simulink model "NolinearObserver"  (R2023b)
settings: Solver=FixedStepDiscrete  StartTime=0.0  StopTime=10  FixedStep=Ts  RelTol=1e-3
values from neighbouring files (symbols this model uses):
  current_bandwidth = 2216.0    [NolinearObserver.sldd]
  flux = 0.0065    [NolinearObserver.sldd]
  Gama = 100000.0    [NolinearObserver.sldd]
  Idq_limit = 10.0    [NolinearObserver.sldd]
  IF_Initial = 30.0    [NolinearObserver.sldd]
  PLL_KI = 20000.0    [NolinearObserver.sldd]
  PLL_KP = 500.0    [NolinearObserver.sldd]
  PMSM_Ls = 8.5E-5    [NolinearObserver.sldd]
  PMSM_Pn = 5.0    [NolinearObserver.sldd]
  PMSM_Rs = 0.03    [NolinearObserver.sldd]
  SPEED_KI = 0.03    [NolinearObserver.sldd]
  SPEED_KP = 0.004    [NolinearObserver.sldd]
  Ts = 0.0001    [NolinearObserver.sldd]
undefined symbols (not defined in the file or in its folder): DiscIntNeverNeededParam
libraries: slpidlib x4, mcbplantlib x1, autolibpmsmexterior x1
settings Model: DataDictionary=NolinearObserver.sldd  NumberOfSteps=50  SnapshotBufferSize=1000  Creator=33595  LastModifiedBy=SkyLin
settings OptimizationCC: DefaultParameterBehavior=Inlined  UseDivisionForNetSlopeComputation=on  GainParamInheritBuiltInType=on  UseFloatMulNetSlope=on  InlineInvariantSignals=on  PassReuseOutputArgsAs=Individual arguments  ZeroExternalMemoryAtStartup=off  ZeroInternalMemoryAtStartup=off  NoFixptDivByZeroProtection=on  EfficientFloat2IntCast=on  LifeSpan=1  OptimizeBlockOrder=speed  DifferentSizesBufferReuse=on  EfficientTunableParamExpr=on
settings DebuggingCC: ParameterOverflowMsg=none  ParameterUnderflowMsg=error  ParameterPrecisionLossMsg=none  ParameterTunabilityLossMsg=error  UnconnectedInputMsg=warning  UnconnectedOutputMsg=warning  UnconnectedLineMsg=warning
settings HardwareCC: ProdBitPerPointer=32  ProdBitPerSizeT=32  ProdBitPerPtrDiffT=32  ProdLargestAtomicInteger=Long  ProdLargestAtomicFloat=Double  ProdWordSize=32  ProdLongLongMode=on  ProdHWDeviceType=ARM Compatible->ARM Cortex-M
settings ModelReferenceCC: EnableRefExpFcnMdlSchedulingChecks=on
settings SFSimCC: MATLABDynamicMemAlloc=off
settings RTWCC: Description=Embedded Coder  SystemTargetFile=ert.tlc  GenCodeOnly=on  TemplateMakefile=ert_default_tmf  RTWUseSimCustomCode=on  DLArmComputeVersion=19.05
settings CodeAppCC: ForceParamTrailComments=on  IgnoreCustomStorageClasses=off  OperatorAnnotations=on  SimulinkDataObjDesc=on  SFDataObjDesc=on  CustomSymbolStrGlobalVar=rt$N$M  CustomSymbolStrType=$N$M  CustomSymbolStrFcn=$N$M$F  CustomSymbolStrMacro=$N$M  InsertBlockDesc=on
settings ERTTargetCC: TargetLangStandard=C99 (ISO)  CodeReplacementLibrary=ARM Cortex-M  GenerateSampleERTMain=on  IncludeMdlTerminateFcn=off  CombineSignalStateStructs=on  SupportComplex=off  SupportNonInlinedSFcns=on  InlinedParameterPlacement=NonHierarchical  ERTCustomFileTemplate=example_file_process.tlc  ERTFilePackagingFormat=CompactWithDataFile  IndentSize=4

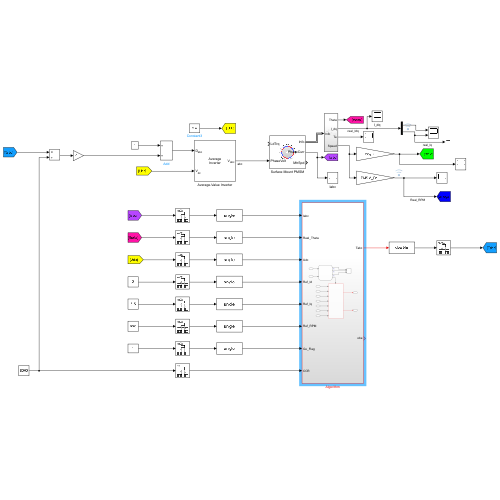
[thumbnail: Simulink's stored preview of the top-level diagram]
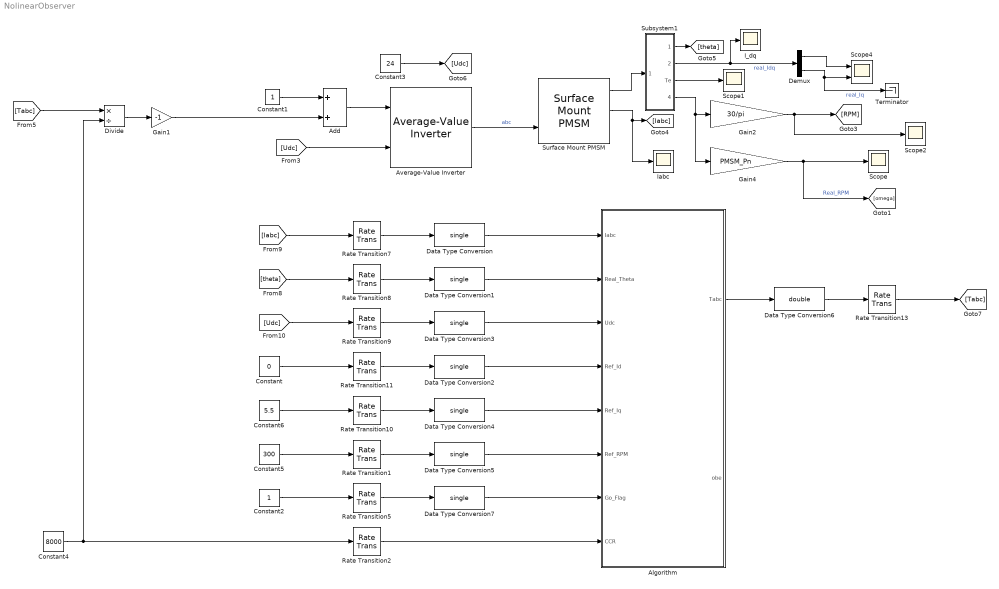
== system NolinearObserver ==
  Add : Sum
  Algorithm : Subsystem
  Average-Value Inverter : mcbplantlib/Average-Value Inverter
  Constant : Constant  Value=0  OutDataTypeStr=single  SampleTime=Ts
  Constant1 : Constant  SampleTime=Ts
  Constant2 : Constant  SampleTime=-1
  Constant3 : Constant  Value=24  SampleTime=Ts
  Constant4 : Constant  Value=8000
  Constant5 : Constant  Value=300
  Constant6 : Constant  Value=5.5
  Data Type Conversion{,1..5,7} (7 alike) : DataTypeConversion  OutDataTypeStr=single  SaturateOnIntegerOverflow=off  RndMeth=Floor
  Data Type Conversion6 : DataTypeConversion  OutDataTypeStr=double  SaturateOnIntegerOverflow=off  RndMeth=Floor
  Demux : Demux  Outputs=2
  Divide : Product  Inputs=*/
  Gain1 : Gain  Gain=-1
  Gain2 : Gain  Gain=30/pi
  Gain4 : Gain  Gain=PMSM_Pn
  I_dq : Scope
  Iabc : Scope
  Rate Transition{1..2,5,8..11,13} (8 alike) : RateTransition  OutPortSampleTime=Ts
  Rate Transition7 : RateTransition
  Scope : Scope
  Scope1 : Scope
  Scope2 : Scope
  Scope4 : Scope  NumInputPorts=2
  Subsystem1 : Subsystem
  Surface Mount PMSM : autolibpmsmexterior/Surface Mount PMSM  port_config=Torque  sim_type=Discrete  Ts=Ts  P=PMSM_Pn  Rs=PMSM_Rs  Ldq_=PMSM_Ls  KConstText=Permanent flux linkage constant (lambda_pm):  lambda_pm=PMSM_flux  Ke=159.9771  Kt=1.323  mechanical=[0.0027, 0.0065, 0]  idq0=[0 0]  theta_init=1  omega_init=0  KConst=PMSM_flux  lambda_pm_calc=PMSM_flux  RefBlkName='autolibpmsmexterior/Surface Mount PMSM'  aMode=5  Ldq="[0.0017      0.0017]"
  Terminator : Terminator
  wires:
  Constant3/1 -> [Udc]
  Subsystem1/1(Theta) -> [theta]
  Subsystem1/2(I_dq) -> Demux/1, I_dq/1  "real_Idq"
  Subsystem1/3(Te) -> Scope1/1
  Subsystem1/4(Speed) -> Gain4/1, Gain2/1
  Average-Value Inverter/1 -> Surface Mount PMSM/2  "abc"
  Surface Mount PMSM/1 -> Subsystem1/1(Info)
  Surface Mount PMSM/2 -> Iabc/1, [Iabc]
  [Udc] -> Average-Value Inverter/2
  Gain2/1 -> Scope2/1, [RPM]
  Gain4/1 -> [omega], Scope/1  "Real_RPM"
  Demux/2 -> Scope4/2, Terminator/1  "real_Iq"
  Data Type Conversion2/1 -> Algorithm/4(Ref_Id)
  [Udc] -> Rate Transition9/1
  Rate Transition13/1 -> [Tabc]
  [Iabc] -> Rate Transition7/1
  Rate Transition10/1 -> Data Type Conversion4/1
  Algorithm/1(Tabc) -> Data Type Conversion6/1
  Data Type Conversion1/1 -> Algorithm/2(Real_Theta)
  Data Type Conversion/1 -> Algorithm/1(Iabc)
  Rate Transition11/1 -> Data Type Conversion2/1
  [theta] -> Rate Transition8/1
  Rate Transition7/1 -> Data Type Conversion/1
  Data Type Conversion6/1 -> Rate Transition13/1
  Rate Transition8/1 -> Data Type Conversion1/1
  Constant/1 -> Rate Transition11/1
  Data Type Conversion4/1 -> Algorithm/5(Ref_Iq)
  Rate Transition9/1 -> Data Type Conversion3/1
  Data Type Conversion3/1 -> Algorithm/3(Udc)
  Add/1 -> Average-Value Inverter/1
  Constant1/1 -> Add/1
  Demux/1 -> Scope4/1
  Rate Transition1/1 -> Data Type Conversion5/1
  Data Type Conversion5/1 -> Algorithm/6(Ref_RPM)
  Constant2/1 -> Rate Transition5/1
  Rate Transition5/1 -> Data Type Conversion7/1
  Data Type Conversion7/1 -> Algorithm/7(Go_Flag)
  Constant6/1 -> Rate Transition10/1
  Constant5/1 -> Rate Transition1/1
  Constant4/1 -> Divide/2, Rate Transition2/1
  Divide/1 -> Gain1/1
  [Tabc] -> Divide/1
  Gain1/1 -> Add/2
  Rate Transition2/1 -> Algorithm/8(CCR)

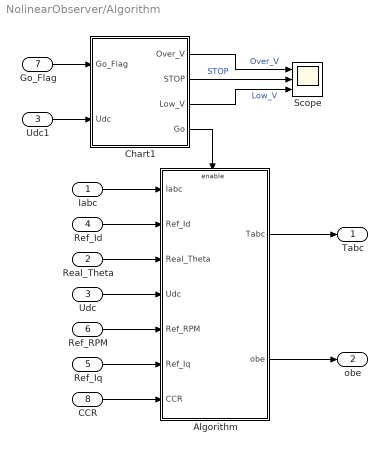
== system NolinearObserver/Algorithm ==
  Iabc : Inport  OutDataTypeStr=single
  Real_Theta : Inport  Port=2  OutDataTypeStr=single
  Udc : Inport  Port=3  OutDataTypeStr=single
  Ref_Id : Inport  Port=4  OutDataTypeStr=single
  Ref_Iq : Inport  Port=5  OutDataTypeStr=single
  Ref_RPM : Inport  Port=6
  Go_Flag : Inport  Port=7
  CCR : Inport  Port=8
  Algorithm : Subsystem
  Chart1 : Stateflow chart  TreatAsAtomicUnit=on
  Scope : Scope  NumInputPorts=3
  Udc1 : InportShadow  Port=3  OutDataTypeStr=single
  Tabc : Outport  OutDataTypeStr=single
  obe : Outport  Port=2
  wires:
  Iabc/1 -> Algorithm/1(Iabc)
  Ref_Id/1 -> Algorithm/2(Ref_Id)
  Real_Theta/1 -> Algorithm/3(Real_Theta)
  Udc/1 -> Algorithm/4(Udc)
  Ref_RPM/1 -> Algorithm/5(Ref_RPM)
  Ref_Iq/1 -> Algorithm/6(Ref_Iq)
  Algorithm/1(Tabc) -> Tabc/1
  Chart1/1(Over_V) -> Scope/1  "Over_V"
  Chart1/2(STOP) -> Scope/2  "STOP"
  Chart1/3(Low_V) -> Scope/3  "Low_V"
  Udc1/1 -> Chart1/2(Udc)
  Go_Flag/1 -> Chart1/1(Go_Flag)
  Chart1/4(Go) -> Algorithm/Enable
  Algorithm/2(obe) -> obe/1
  CCR/1 -> Algorithm/7(CCR)

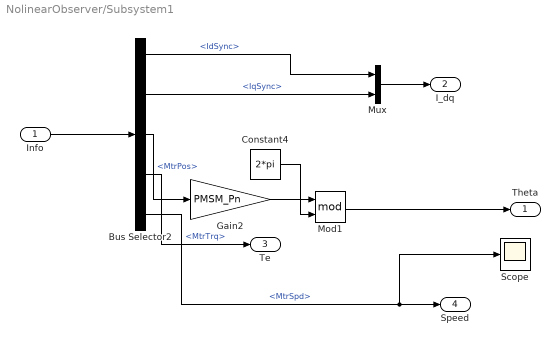
== system NolinearObserver/Subsystem1 ==
  Info : Inport
  Bus Selector2 : BusSelector  OutputSignals=IdSync,IqSync,MtrPos,MtrTrq,MtrSpd
  Constant4 : Constant  Value=2*pi  SampleTime=-1
  Gain2 : Gain  Gain=PMSM_Pn
  Mod1 : Math  Operator=mod
  Mux : Mux  Inputs=2
  Scope : Scope
  Theta : Outport
  I_dq : Outport  Port=2
  Te : Outport  Port=3
  Speed : Outport  Port=4
  wires:
  Bus Selector2/2 -> Mux/2  "<IqSync>"
  Gain2/1 -> Mod1/1
  Mod1/1 -> Theta/1
  Bus Selector2/1 -> Mux/1  "<IdSync>"
  Constant4/1 -> Mod1/2
  Info/1 -> Bus Selector2/1
  Bus Selector2/3 -> Gain2/1  "<MtrPos>"
  Mux/1 -> I_dq/1
  Bus Selector2/4 -> Te/1  "<MtrTrq>"
  Bus Selector2/5 -> Scope/1, Speed/1  "<MtrSpd>"

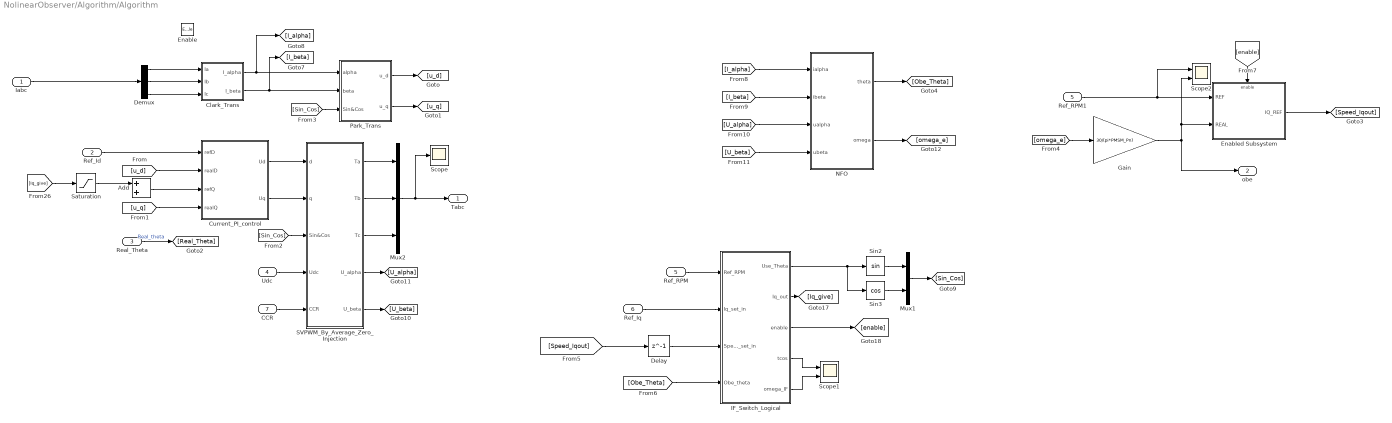
== system NolinearObserver/Algorithm/Algorithm ==
  Iabc : Inport
  Ref_Id : Inport  Port=2
  Real_Theta : Inport  Port=3
  Udc : Inport  Port=4
  Ref_RPM : Inport  Port=5
  Ref_Iq : Inport  Port=6
  CCR : Inport  Port=7
  Enable : EnablePort
  Add : Sum  OutDataTypeStr=single
  Clark_Trans : Subsystem  TreatAsAtomicUnit=on
      settings: RTWFcnNameOpts=Use subsystem name
  Current_PI_control : Subsystem  TreatAsAtomicUnit=on
      settings: RTWFcnNameOpts=Use subsystem name
  Delay : Delay  DelayLength=1
  Demux : Demux  Outputs=3
  Enabled Subsystem : Subsystem  TreatAsAtomicUnit=on
  Gain : Gain  Gain=30/(pi*PMSM_Pn)
  IF_Switch_Logical : Stateflow chart  TreatAsAtomicUnit=on
  Mux1 : Mux  Inputs=2
  Mux2 : Mux  Inputs=3
  NFO : Subsystem
  Park_Trans : Subsystem  TreatAsAtomicUnit=on
      settings: RTWFcnNameOpts=Use subsystem name
  Ref_RPM1 : InportShadow  Port=5
  SVPWM_By_Average_Zero_Injection : Subsystem  TreatAsAtomicUnit=on
  Saturation : Saturate  UpperLimit=Idq_limit  LowerLimit=-Idq_limit  OutDataTypeStr=single
  Scope : Scope
  Scope1 : Scope  NumInputPorts=2
  Scope2 : Scope  NumInputPorts=2
  Sin2 : Trigonometry
  Sin3 : Trigonometry  Operator=cos
  Tabc : Outport
  obe : Outport  Port=2
  wires:
  Sin3/1 -> Mux1/2
  Sin2/1 -> Mux1/1
  Add/1 -> Current_PI_control/3(refQ)
  Iabc/1 -> Demux/1
  [Sin_Cos] -> Park_Trans/3(Sin&Cos)
  Clark_Trans/2(I_beta) -> [I_beta], Park_Trans/2(beta)
  Demux/3 -> Clark_Trans/3(Ic)
  Clark_Trans/1(I_alpha) -> [I_alpha], Park_Trans/1(alpha)
  Park_Trans/2(u_q) -> [u_q]
  SVPWM_By_Average_Zero_Injection/2(Tb) -> Mux2/2
  SVPWM_By_Average_Zero_Injection/3(Tc) -> Mux2/3
  SVPWM_By_Average_Zero_Injection/1(Ta) -> Mux2/1
  [u_q] -> Current_PI_control/4(realQ)
  Demux/2 -> Clark_Trans/2(Ib)
  [Sin_Cos] -> SVPWM_By_Average_Zero_Injection/3(Sin&Cos)
  SVPWM_By_Average_Zero_Injection/5(U_beta) -> [U_beta]
  Park_Trans/1(u_d) -> [u_d]
  [u_d] -> Current_PI_control/2(realD)
  Demux/1 -> Clark_Trans/1(Ia)
  [Iq_give] -> Saturation/1
  SVPWM_By_Average_Zero_Injection/4(U_alpha) -> [U_alpha]
  Current_PI_control/1(Ud) -> SVPWM_By_Average_Zero_Injection/1(d)
  Saturation/1 -> Add/1
  Mux2/1 -> Scope/1, Tabc/1
  Current_PI_control/2(Uq) -> SVPWM_By_Average_Zero_Injection/2(q)
  Ref_Id/1 -> Current_PI_control/1(refD)
  Mux1/1 -> [Sin_Cos]
  Real_Theta/1 -> [Real_Theta]  "Real_theta"
  Udc/1 -> SVPWM_By_Average_Zero_Injection/4(Udc)
  Ref_RPM/1 -> IF_Switch_Logical/1(Ref_RPM)
  IF_Switch_Logical/1(Use_Theta) -> Sin3/1, Sin2/1
  Ref_Iq/1 -> IF_Switch_Logical/2(Iq_set_in)
  IF_Switch_Logical/2(Iq_out) -> [Iq_give]
  IF_Switch_Logical/3(enable) -> [enable]
  IF_Switch_Logical/4(tcos) -> Scope1/1
  IF_Switch_Logical/5(omega_IF) -> Scope1/2
  Enabled Subsystem/1(IQ_REF) -> [Speed_Iqout]
  [enable] -> Enabled Subsystem/Enable
  Ref_RPM1/1 -> Scope2/1, Enabled Subsystem/1(REF)
  Gain/1 -> Scope2/2, Enabled Subsystem/2(REAL), obe/1
  CCR/1 -> SVPWM_By_Average_Zero_Injection/5(CCR)
  [I_alpha] -> NFO/1(ialpha)
  [I_beta] -> NFO/2(ibeta)
  [U_alpha] -> NFO/3(ualpha)
  [U_beta] -> NFO/4(ubeta)
  [omega_e] -> Gain/1
  [Obe_Theta] -> IF_Switch_Logical/4(Obe_theta)
  [Speed_Iqout] -> Delay/1
  Delay/1 -> IF_Switch_Logical/3(Speed_set_in)
  NFO/1(theta) -> [Obe_Theta]
  NFO/2(omega) -> [omega_e]

== system NolinearObserver/Algorithm/Chart1/Low_judge ==
  Input : Inport  OutDataTypeStr=single  PortDimensions=1
  f : TriggerPort  TriggerType=function-call  VariantControl=(inherit)
      settings: CopyFcn=Stateflow.SLINSF.SimulinkMan.removeBlockPreDeleteFcn  PreDeleteFcn=Stateflow.SLINSF.SimulinkMan.unsafePredeleteFcn
  Data Type Conversion : DataTypeConversion  OutDataTypeStr=boolean  SaturateOnIntegerOverflow=off  RndMeth=Floor
  Data Type Conversion1 : DataTypeConversion  OutDataTypeStr=single  SaturateOnIntegerOverflow=off  RndMeth=Floor
  NOR : Logic  Operator=NOT  IconShape=distinctive  OutDataTypeStr=boolean
  Relay : Relay  OnSwitchValue=20  OffSwitchValue=18  OutDataTypeStr=single
  Out : Outport  OutDataTypeStr=single
  wires:
  Input/1 -> Relay/1
  Relay/1 -> Data Type Conversion/1
  NOR/1 -> Data Type Conversion1/1
  Data Type Conversion/1 -> NOR/1
  Data Type Conversion1/1 -> Out/1

== system NolinearObserver/Algorithm/Chart1/Over_judge ==
  Input : Inport  OutDataTypeStr=single  PortDimensions=1
  f : TriggerPort  TriggerType=function-call  VariantControl=(inherit)
      settings: CopyFcn=Stateflow.SLINSF.SimulinkMan.removeBlockPreDeleteFcn  PreDeleteFcn=Stateflow.SLINSF.SimulinkMan.unsafePredeleteFcn
  Relay : Relay  OnSwitchValue=28  OffSwitchValue=25  OutDataTypeStr=single
  Out : Outport  OutDataTypeStr=single
  wires:
  Input/1 -> Relay/1
  Relay/1 -> Out/1

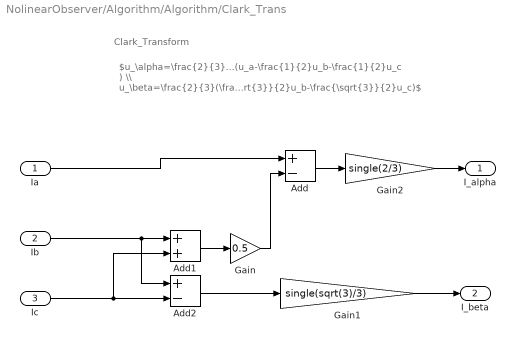
== system NolinearObserver/Algorithm/Algorithm/Clark_Trans ==
  note: $u_\alpha=\frac{2}{3}(u_a-\frac{1}{2}u_b-\frac{1}{2}u_c ) \\ u_\beta=\frac{2}{3}(\frac{\sqrt{3}}{2}u_b-\frac{\sqrt{3}}{2}u_c)$
  note: Clark_Transform
  Ia : Inport  OutDataTypeStr=single
  Ib : Inport  Port=2  OutDataTypeStr=single
  Ic : Inport  Port=3  OutDataTypeStr=single
  Add : Sum  Inputs=+-  OutDataTypeStr=single
  Add1 : Sum  OutDataTypeStr=single
  Add2 : Sum  Inputs=+-  OutDataTypeStr=single
  Gain : Gain  Gain=0.5  OutDataTypeStr=single
  Gain1 : Gain  Gain=single(sqrt(3)/3)  OutDataTypeStr=single
  Gain2 : Gain  Gain=single(2/3)  OutDataTypeStr=single
  I_alpha : Outport  OutDataTypeStr=single
  I_beta : Outport  Port=2
  wires:
  Ia/1 -> Add/1
  Gain/1 -> Add/2
  Ib/1 -> Add1/1, Add2/1
  Ic/1 -> Add1/2, Add2/2
  Add2/1 -> Gain1/1
  Add1/1 -> Gain/1
  Add/1 -> Gain2/1
  Gain2/1 -> I_alpha/1
  Gain1/1 -> I_beta/1

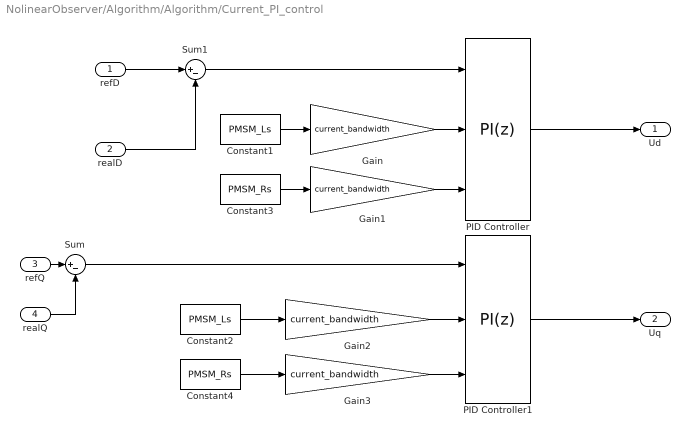
== system NolinearObserver/Algorithm/Algorithm/Current_PI_control ==
  refD : Inport  OutDataTypeStr=single
  realD : Inport  Port=2  OutDataTypeStr=single
  refQ : Inport  Port=3  OutDataTypeStr=single
  realQ : Inport  Port=4  OutDataTypeStr=single
  Constant1 : Constant  Value=PMSM_Ls  OutDataTypeStr=single  SampleTime=Ts
  Constant2 : Constant  Value=PMSM_Ls  OutDataTypeStr=single  SampleTime=Ts
  Constant3 : Constant  Value=PMSM_Rs  OutDataTypeStr=single  SampleTime=Ts
  Constant4 : Constant  Value=PMSM_Rs  OutDataTypeStr=single  SampleTime=Ts
  Gain{,1..3} (4 alike) : Gain  Gain=current_bandwidth  OutDataTypeStr=single
  PID Controller : slpidlib/PID Controller  Controller=PI  Form=Parallel  TimeDomain=Discrete-time  UseExternalTs=off  SampleTime=Ts  IntegratorMethod=Forward Euler  FilterMethod=Forward Euler  ControllerParametersSource=external  P=1  I=1  UseKiTs=off  D=0  N=100  UseFilter=on  TunerSelectOption=Transfer Function Based (PID Tuner App)  ZeroCross=off  InitialConditionSource=internal  InitialConditionForIntegrator=0  InitialConditionForFilter=0  DifferentiatorICPrevScaledInput=0  ExternalReset=none  TrackingMode=off  Kt=1  LimitOutput=on  SatLimitsSource=internal  UpperSaturationLimit=Idq_limit  LowerSaturationLimit=-Idq_limit  LinearizeAsGain=off  AntiWindupMode=none  Kb=1  LimitIntegrator=off  UpperIntegratorSaturationLimit=inf  LowerIntegratorSaturationLimit=-inf  POutMin=[]  POutMax=[]  IOutMin=[]  IOutMax=[]  DOutMin=[]  DOutMax=[]  NOutMin=[]  NOutMax=[]  SumOutMin=[]  SumOutMax=[]  SaturationOutMin=[]  SaturationOutMax=[]  PParamMin=[]  PParamMax=[]  IParamMin=[]  IParamMax=[]  DParamMin=[]  DParamMax=[]  NParamMin=[]  NParamMax=[]  KbParamMin=[]  KbParamMax=[]  KtParamMin=[]  KtParamMax=[]  KbOutMin=[]  KbOutMax=[]  KtOutMin=[]  KtOutMax=[]  IntegratorOutMin=[]  IntegratorOutMax=[]  FilterOutMin=[]  FilterOutMax=[]  SumI1OutMin=[]  SumI1OutMax=[]  SumI2OutMin=[]  SumI2OutMax=[]  SumI3OutMin=[]  SumI3OutMax=[]  SumI4OutMin=[]  SumI4OutMax=[]  SumDOutMin=[]  SumDOutMax=[]  DifferentiatorOutMin=[]  DifferentiatorOutMax=[]  FilterDiffOutCoefMin=[]  FilterDiffOutCoefMax=[]  ReciprocalOutMin=[]  ReciprocalOutMax=[]  SumDenOutMin=[]  SumDenOutMax=[]  SumNumOutMin=[]  SumNumOutMax=[]  DivideOutMin=[]  DivideOutMax=[]  UdiffTsProdOutMin=[]  UdiffTsProdOutMax=[]  NTsProdOutMin=[]  NTsProdOutMax=[]  UintegralTsProdOutMin=[]  UintegralTsProdOutMax=[]  UngainTsProdOutMin=[]  UngainTsProdOutMax=[]  ClampingZeroOutDataTypeStr=Inherit: Inherit via back propagation  ClampingZeroOutMin=[]  ClampingZeroOutMax=[]  FilterDenConstantOutDataTypeStr=Inherit: Inherit via back propagation  FilterDenConstantOutMin=[]  FilterDenConstantOutMax=[]  PCopyOutDataTypeStr=Inherit: Inherit via back propagation  PCopyOutMin=[]  PCopyOutMax=[]  NCopyOutDataTypeStr=Inherit: Inherit via back propagation  NCopyOutMin=[]  NCopyOutMax=[]  IntegratorContinuousStateAttributes=''  IntegratorStateMustResolveToSignalObject=off  IntegratorRTWStateStorageClass=Auto  FilterContinuousStateAttributes=''  FilterStateMustResolveToSignalObject=off  FilterRTWStateStorageClass=Auto  ParallelPVariant=ExternalParameters  IdealPVariant=Disabled  IVariant=ExternalParameters  DVariant=Disabled  IntegratorVariant=Discrete  SatVariant=Enabled  AWVariant=Passthrough  PCopyVariant=Disabled  TRVariant=Disabled  FdbkBlocksVariant=Forward  IdealPFdbkVariant=Disabled  SatFdbkVariant=Disabled  DerivativeFilterVariant=Disabled  NVariant=Disabled  NCopyVariant=Disabled_SignalSpec  FilterICVariant=Disabled  IntegratorICVariant=InternalICs  ExternalResetVariant=Disabled  TRSumVariant=Passthrough  SumFdbkVariant=Disabled  SumVariant=Sum_PI  TsampFilterVariant=InternalTs  TsampNgainVariant=Passthrough  TsampIntegralVariant=Disabled_SignalSpec  ExternalSaturationOutDataTypeStr=Inherit: Same as second input
  PID Controller1 : slpidlib/PID Controller  Controller=PI  Form=Parallel  TimeDomain=Discrete-time  UseExternalTs=off  SampleTime=Ts  IntegratorMethod=Forward Euler  FilterMethod=Forward Euler  ControllerParametersSource=external  P=1  I=1  UseKiTs=off  D=0  N=100  UseFilter=on  TunerSelectOption=Transfer Function Based (PID Tuner App)  ZeroCross=off  InitialConditionSource=internal  InitialConditionForIntegrator=0  InitialConditionForFilter=0  DifferentiatorICPrevScaledInput=0  ExternalReset=none  TrackingMode=off  Kt=1  LimitOutput=on  SatLimitsSource=internal  UpperSaturationLimit=Idq_limit  LowerSaturationLimit=-Idq_limit  LinearizeAsGain=off  AntiWindupMode=none  Kb=1  LimitIntegrator=off  UpperIntegratorSaturationLimit=inf  LowerIntegratorSaturationLimit=-inf  POutMin=[]  POutMax=[]  IOutMin=[]  IOutMax=[]  DOutMin=[]  DOutMax=[]  NOutMin=[]  NOutMax=[]  SumOutMin=[]  SumOutMax=[]  SaturationOutMin=[]  SaturationOutMax=[]  PParamMin=[]  PParamMax=[]  IParamMin=[]  IParamMax=[]  DParamMin=[]  DParamMax=[]  NParamMin=[]  NParamMax=[]  KbParamMin=[]  KbParamMax=[]  KtParamMin=[]  KtParamMax=[]  KbOutMin=[]  KbOutMax=[]  KtOutMin=[]  KtOutMax=[]  IntegratorOutMin=[]  IntegratorOutMax=[]  FilterOutMin=[]  FilterOutMax=[]  SumI1OutMin=[]  SumI1OutMax=[]  SumI2OutMin=[]  SumI2OutMax=[]  SumI3OutMin=[]  SumI3OutMax=[]  SumI4OutMin=[]  SumI4OutMax=[]  SumDOutMin=[]  SumDOutMax=[]  DifferentiatorOutMin=[]  DifferentiatorOutMax=[]  FilterDiffOutCoefMin=[]  FilterDiffOutCoefMax=[]  ReciprocalOutMin=[]  ReciprocalOutMax=[]  SumDenOutMin=[]  SumDenOutMax=[]  SumNumOutMin=[]  SumNumOutMax=[]  DivideOutMin=[]  DivideOutMax=[]  UdiffTsProdOutMin=[]  UdiffTsProdOutMax=[]  NTsProdOutMin=[]  NTsProdOutMax=[]  UintegralTsProdOutMin=[]  UintegralTsProdOutMax=[]  UngainTsProdOutMin=[]  UngainTsProdOutMax=[]  ClampingZeroOutDataTypeStr=Inherit: Inherit via back propagation  ClampingZeroOutMin=[]  ClampingZeroOutMax=[]  FilterDenConstantOutDataTypeStr=Inherit: Inherit via back propagation  FilterDenConstantOutMin=[]  FilterDenConstantOutMax=[]  PCopyOutDataTypeStr=Inherit: Inherit via back propagation  PCopyOutMin=[]  PCopyOutMax=[]  NCopyOutDataTypeStr=Inherit: Inherit via back propagation  NCopyOutMin=[]  NCopyOutMax=[]  IntegratorContinuousStateAttributes=''  IntegratorStateMustResolveToSignalObject=off  IntegratorRTWStateStorageClass=Auto  FilterContinuousStateAttributes=''  FilterStateMustResolveToSignalObject=off  FilterRTWStateStorageClass=Auto  ParallelPVariant=ExternalParameters  IdealPVariant=Disabled  IVariant=ExternalParameters  DVariant=Disabled  IntegratorVariant=Discrete  SatVariant=Enabled  AWVariant=Passthrough  PCopyVariant=Disabled  TRVariant=Disabled  FdbkBlocksVariant=Forward  IdealPFdbkVariant=Disabled  SatFdbkVariant=Disabled  DerivativeFilterVariant=Disabled  NVariant=Disabled  NCopyVariant=Disabled_SignalSpec  FilterICVariant=Disabled  IntegratorICVariant=InternalICs  ExternalResetVariant=Disabled  TRSumVariant=Passthrough  SumFdbkVariant=Disabled  SumVariant=Sum_PI  TsampFilterVariant=InternalTs  TsampNgainVariant=Passthrough  TsampIntegralVariant=Disabled_SignalSpec  ExternalSaturationOutDataTypeStr=Inherit: Same as second input
  Sum : Sum  Inputs=|+-  OutDataTypeStr=single
  Sum1 : Sum  Inputs=|+-  OutDataTypeStr=single
  Ud : Outport  OutDataTypeStr=single
  Uq : Outport  Port=2  OutDataTypeStr=single
  wires:
  realD/1 -> Sum1/2
  realQ/1 -> Sum/2
  PID Controller1/1 -> Uq/1
  PID Controller/1 -> Ud/1
  Sum/1 -> PID Controller1/1
  Sum1/1 -> PID Controller/1
  refD/1 -> Sum1/1
  refQ/1 -> Sum/1
  Constant2/1 -> Gain2/1
  Gain3/1 -> PID Controller1/3
  Gain/1 -> PID Controller/2
  Gain2/1 -> PID Controller1/2
  Constant1/1 -> Gain/1
  Constant4/1 -> Gain3/1
  Gain1/1 -> PID Controller/3
  Constant3/1 -> Gain1/1

== system NolinearObserver/Algorithm/Algorithm/Enabled Subsystem ==
  REF : Inport
  REAL : Inport  Port=2
  Enable : EnablePort
  PID Controller : slpidlib/PID Controller  Controller=PI  Form=Parallel  TimeDomain=Discrete-time  UseExternalTs=off  SampleTime=Ts  IntegratorMethod=Forward Euler  FilterMethod=Forward Euler  ControllerParametersSource=internal  P=SPEED_KP  I=SPEED_KI  UseKiTs=off  D=0  N=100  UseFilter=on  TunerSelectOption=Transfer Function Based (PID Tuner App)  InitialConditionSource=internal  InitialConditionForIntegrator=0  InitialConditionForFilter=0  DifferentiatorICPrevScaledInput=0  ExternalReset=none  TrackingMode=off  Kt=1  LimitOutput=on  SatLimitsSource=internal  UpperSaturationLimit=10  LowerSaturationLimit=-10  LinearizeAsGain=on  AntiWindupMode=none  Kb=1  LimitIntegrator=off  UpperIntegratorSaturationLimit=inf  LowerIntegratorSaturationLimit=-inf  POutMin=[]  POutMax=[]  IOutMin=[]  IOutMax=[]  DOutMin=[]  DOutMax=[]  NOutMin=[]  NOutMax=[]  SumOutMin=[]  SumOutMax=[]  SaturationOutMin=[]  SaturationOutMax=[]  PParamMin=[]  PParamMax=[]  IParamMin=[]  IParamMax=[]  DParamMin=[]  DParamMax=[]  NParamMin=[]  NParamMax=[]  KbParamMin=[]  KbParamMax=[]  KtParamMin=[]  KtParamMax=[]  KbOutMin=[]  KbOutMax=[]  KtOutMin=[]  KtOutMax=[]  IntegratorOutMin=[]  IntegratorOutMax=[]  FilterOutMin=[]  FilterOutMax=[]  SumI1OutMin=[]  SumI1OutMax=[]  SumI2OutMin=[]  SumI2OutMax=[]  SumI3OutMin=[]  SumI3OutMax=[]  SumI4OutMin=[]  SumI4OutMax=[]  SumDOutMin=[]  SumDOutMax=[]  DifferentiatorOutMin=[]  DifferentiatorOutMax=[]  FilterDiffOutCoefMin=[]  FilterDiffOutCoefMax=[]  ReciprocalOutMin=[]  ReciprocalOutMax=[]  SumDenOutMin=[]  SumDenOutMax=[]  SumNumOutMin=[]  SumNumOutMax=[]  DivideOutMin=[]  DivideOutMax=[]  UdiffTsProdOutMin=[]  UdiffTsProdOutMax=[]  NTsProdOutMin=[]  NTsProdOutMax=[]  UintegralTsProdOutMin=[]  UintegralTsProdOutMax=[]  UngainTsProdOutMin=[]  UngainTsProdOutMax=[]  ClampingZeroOutDataTypeStr=Inherit: Inherit via back propagation  ClampingZeroOutMin=[]  ClampingZeroOutMax=[]  FilterDenConstantOutDataTypeStr=Inherit: Inherit via back propagation  FilterDenConstantOutMin=[]  FilterDenConstantOutMax=[]  PCopyOutDataTypeStr=Inherit: Inherit via back propagation  PCopyOutMin=[]  PCopyOutMax=[]  NCopyOutDataTypeStr=Inherit: Inherit via back propagation  NCopyOutMin=[]  NCopyOutMax=[]  IntegratorContinuousStateAttributes=''  IntegratorStateMustResolveToSignalObject=off  IntegratorRTWStateStorageClass=Auto  FilterContinuousStateAttributes=''  FilterStateMustResolveToSignalObject=off  FilterRTWStateStorageClass=Auto  ParallelPVariant=InternalParameters  IdealPVariant=Disabled  IVariant=InternalParameters  DVariant=Disabled  IntegratorVariant=Discrete  SatVariant=Enabled  AWVariant=Passthrough  PCopyVariant=Disabled  TRVariant=Disabled  FdbkBlocksVariant=Forward  IdealPFdbkVariant=Disabled  SatFdbkVariant=Disabled  DerivativeFilterVariant=Disabled  NVariant=Disabled  NCopyVariant=Disabled_SignalSpec  FilterICVariant=Disabled  IntegratorICVariant=InternalICs  ExternalResetVariant=Disabled  TRSumVariant=Passthrough  SumFdbkVariant=Disabled  SumVariant=Sum_PI  TsampFilterVariant=InternalTs  TsampNgainVariant=Passthrough  TsampIntegralVariant=Disabled_SignalSpec  ExternalSaturationOutDataTypeStr=Inherit: Same as second input
  Sum : Sum  Inputs=|+-
  IQ_REF : Outport
  wires:
  REF/1 -> Sum/1
  REAL/1 -> Sum/2
  Sum/1 -> PID Controller/1
  PID Controller/1 -> IQ_REF/1

== system NolinearObserver/Algorithm/Algorithm/IF_Switch_Logical/Forward_theta ==
  direction : Inport  OutDataTypeStr=single  PortDimensions=1
  f : TriggerPort  TriggerType=function-call  VariantControl=(inherit)
      settings: CopyFcn=Stateflow.SLINSF.SimulinkMan.removeBlockPreDeleteFcn  PreDeleteFcn=Stateflow.SLINSF.SimulinkMan.unsafePredeleteFcn
  Constant : Constant  Value=IF_Initial  OutDataTypeStr=single
  Discrete-Time Integrator : DiscreteIntegrator  SampleTime=-1  ICPrevOutput=DiscIntNeverNeededParam  ICPrevScaledInput=DiscIntNeverNeededParam
  Product : Product
  integrator : Subsystem
  IF_theta : Outport  OutDataTypeStr=single
  IF_omega : Outport  Port=2  OutDataTypeStr=single
  wires:
  Constant/1 -> Discrete-Time Integrator/1
  integrator/1(y(k-1)) -> IF_theta/1
  direction/1 -> Product/2
  Discrete-Time Integrator/1 -> Product/1
  Product/1 -> IF_omega/1, integrator/1(x(k))

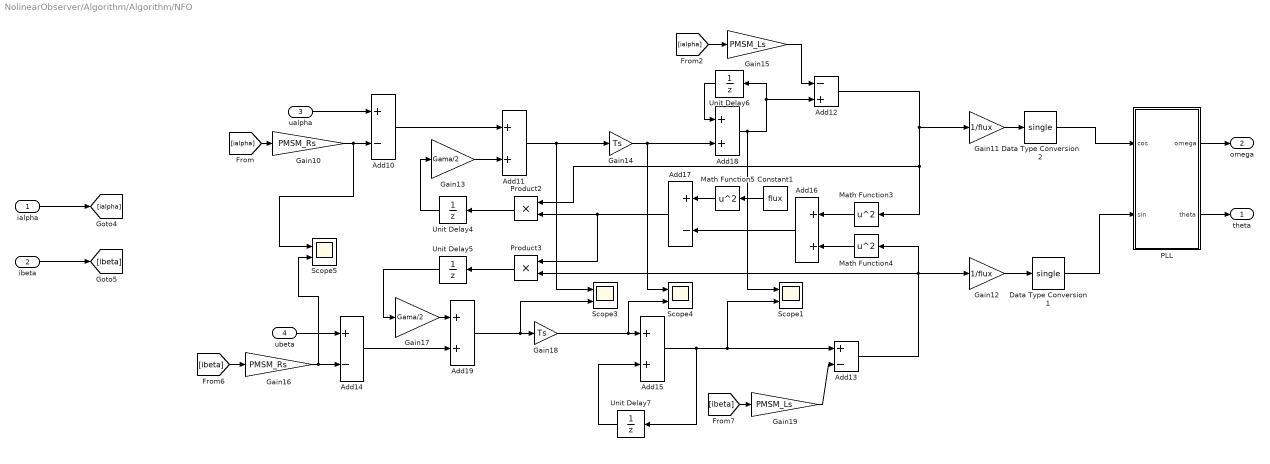
== system NolinearObserver/Algorithm/Algorithm/NFO ==
  ialpha : Inport
  ibeta : Inport  Port=2
  ualpha : Inport  Port=3
  ubeta : Inport  Port=4
  Add{10,13..14,17} (4 alike) : Sum  Inputs=+-
  Add{11,15..16,18..19} (5 alike) : Sum
  Add12 : Sum  Inputs=-+
  Constant1 : Constant  Value=flux
  Data Type Conversion1 : DataTypeConversion  OutDataTypeStr=single  SaturateOnIntegerOverflow=off  RndMeth=Floor
  Data Type Conversion2 : DataTypeConversion  OutDataTypeStr=single  SaturateOnIntegerOverflow=off  RndMeth=Floor
  Gain10 : Gain  Gain=PMSM_Rs
  Gain11 : Gain  Gain=1/flux
  Gain12 : Gain  Gain=1/flux
  Gain13 : Gain  Gain=Gama/2
  Gain14 : Gain  Gain=Ts
  Gain15 : Gain  Gain=PMSM_Ls
  Gain16 : Gain  Gain=PMSM_Rs
  Gain17 : Gain  Gain=Gama/2
  Gain18 : Gain  Gain=Ts
  Gain19 : Gain  Gain=PMSM_Ls
  Math Function3 : Math  Operator=square
  Math Function4 : Math  Operator=square
  Math Function5 : Math  Operator=square
  PLL : Subsystem
  Product2 : Product
  Product3 : Product
  Scope{1,3..5} (4 alike) : Scope  NumInputPorts=2
  Unit Delay{4..7} (4 alike) : UnitDelay  SampleTime=-1  HasFrameUpgradeWarning=on
  theta : Outport  OutDataTypeStr=single
  omega : Outport  Port=2  OutDataTypeStr=single
  wires:
  Gain15/1 -> Add12/1
  Gain17/1 -> Add19/1
  Add17/1 -> Product3/1, Product2/2
  Product3/1 -> Unit Delay5/1
  Add15/1 -> Scope1/2, Add13/1, Unit Delay7/1
  Add19/1 -> Scope3/2, Gain18/1
  [ialpha] -> Gain15/1
  Add13/1 -> Product3/2, Math Function4/1, Gain12/1
  Product2/1 -> Unit Delay4/1
  Gain14/1 -> Scope4/1, Add18/2
  Gain19/1 -> Add13/2
  Add12/1 -> Product2/1, Math Function3/1, Gain11/1
  Unit Delay6/1 -> Add18/1
  ibeta/1 -> [ibeta]
  Gain16/1 -> Scope5/2, Add14/2
  Gain13/1 -> Add11/2
  Add14/1 -> Add19/2
  Unit Delay4/1 -> Gain13/1
  Add10/1 -> Add11/1
  Add16/1 -> Add17/2
  Math Function5/1 -> Add17/1
  [ibeta] -> Gain19/1
  Constant1/1 -> Math Function5/1
  Add18/1 -> Scope1/1, Unit Delay6/1, Add12/2
  Unit Delay7/1 -> Add15/2
  [ibeta] -> Gain16/1
  Math Function4/1 -> Add16/2
  Unit Delay5/1 -> Gain17/1
  Gain18/1 -> Scope4/2, Add15/1
  Add11/1 -> Scope3/1, Gain14/1
  Gain10/1 -> Scope5/1, Add10/2
  Math Function3/1 -> Add16/1
  ialpha/1 -> [ialpha]
  ualpha/1 -> Add10/1
  [ialpha] -> Gain10/1
  ubeta/1 -> Add14/1
  Gain11/1 -> Data Type Conversion2/1
  Gain12/1 -> Data Type Conversion1/1
  Data Type Conversion2/1 -> PLL/1(cos)
  Data Type Conversion1/1 -> PLL/2(sin)
  PLL/1(omega) -> omega/1
  PLL/2(theta) -> theta/1

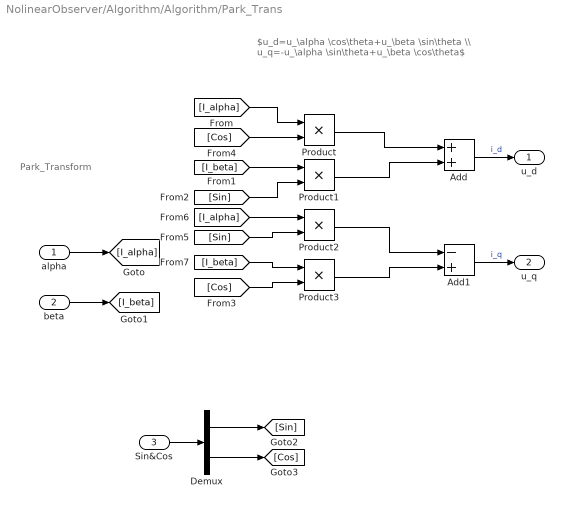
== system NolinearObserver/Algorithm/Algorithm/Park_Trans ==
  note: $u_d=u_\alpha \cos\theta+u_\beta \sin\theta \\ u_q=-u_\alpha \sin\theta+u_\beta \cos\theta$
  note: Park_Transform
  alpha : Inport  OutDataTypeStr=single
  beta : Inport  Port=2  OutDataTypeStr=single
  Sin&Cos : Inport  Port=3  OutDataTypeStr=single
  Add : Sum  OutDataTypeStr=single
  Add1 : Sum  Inputs=-+  OutDataTypeStr=single
  Demux : Demux  Outputs=2
  Product{,1..3} (4 alike) : Product  OutDataTypeStr=single
  u_d : Outport  OutDataTypeStr=single
  u_q : Outport  Port=2  OutDataTypeStr=single
  wires:
  Add1/1 -> u_q/1  "i_q"
  [Cos] -> Product/2
  Product/1 -> Add/1
  Product1/1 -> Add/2
  beta/1 -> [I_beta]
  Add/1 -> u_d/1  "i_d"
  [I_alpha] -> Product/1
  Product3/1 -> Add1/2
  [I_beta] -> Product3/1
  [I_beta] -> Product1/1
  [Sin] -> Product2/2
  Product2/1 -> Add1/1
  [Sin] -> Product1/2
  [I_alpha] -> Product2/1
  alpha/1 -> [I_alpha]
  [Cos] -> Product3/2
  Demux/1 -> [Sin]
  Demux/2 -> [Cos]
  Sin&Cos/1 -> Demux/1

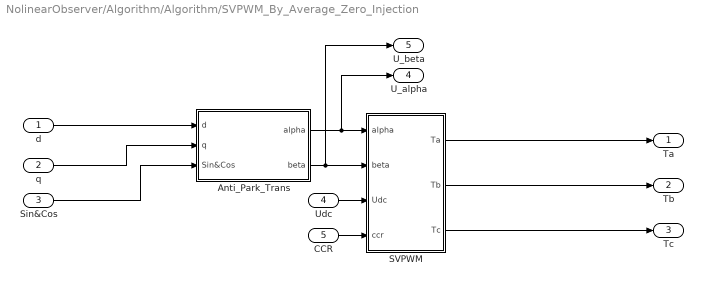
== system NolinearObserver/Algorithm/Algorithm/SVPWM_By_Average_Zero_Injection ==
  d : Inport  OutDataTypeStr=single
  q : Inport  Port=2  OutDataTypeStr=single
  Sin&Cos : Inport  Port=3  OutDataTypeStr=single
  Udc : Inport  Port=4  OutDataTypeStr=single
  CCR : Inport  Port=5
  Anti_Park_Trans : Subsystem
  SVPWM : Subsystem
  Ta : Outport  OutDataTypeStr=single
  Tb : Outport  Port=2  OutDataTypeStr=single
  Tc : Outport  Port=3  OutDataTypeStr=single
  U_alpha : Outport  Port=4  OutDataTypeStr=single
  U_beta : Outport  Port=5  OutDataTypeStr=single
  wires:
  Anti_Park_Trans/1(alpha) -> U_alpha/1, SVPWM/1(alpha)
  q/1 -> Anti_Park_Trans/2(q)
  Anti_Park_Trans/2(beta) -> U_beta/1, SVPWM/2(beta)
  d/1 -> Anti_Park_Trans/1(d)
  Sin&Cos/1 -> Anti_Park_Trans/3(Sin&Cos)
  Udc/1 -> SVPWM/3(Udc)
  SVPWM/1(Ta) -> Ta/1
  SVPWM/2(Tb) -> Tb/1
  SVPWM/3(Tc) -> Tc/1
  CCR/1 -> SVPWM/4(ccr)

== system NolinearObserver/Algorithm/Algorithm/IF_Switch_Logical/Forward_theta/integrator ==
  note: $y(k)=x(k)*T_s+y(k-1)$
  x(k) : Inport  OutDataTypeStr=single
  RangeLimit : Subsystem
  Sum1 : Sum  Inputs=|++  OutDataTypeStr=single
  Ts : Gain  Gain=Ts  OutDataTypeStr=single
  Unit Delay : UnitDelay  SampleTime=-1  HasFrameUpgradeWarning=on
  y(k-1) : Outport  OutDataTypeStr=single
  wires:
  x(k)/1 -> Ts/1
  Ts/1 -> Sum1/1
  Sum1/1 -> RangeLimit/1(In)  "y(k)"
  Unit Delay/1 -> y(k-1)/1, Sum1/2
  RangeLimit/1(Theta) -> Unit Delay/1

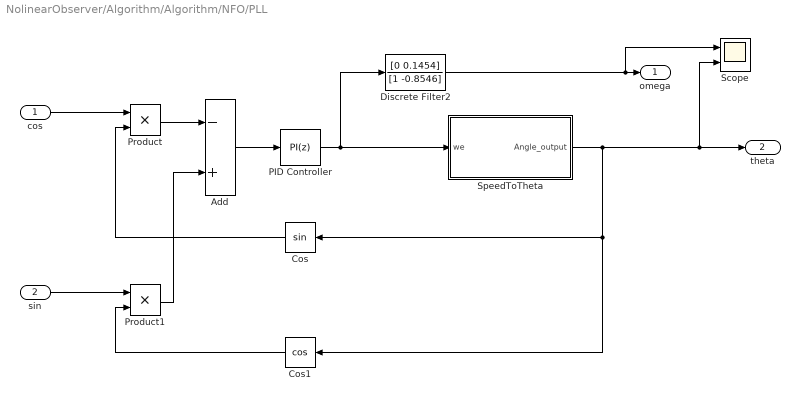
== system NolinearObserver/Algorithm/Algorithm/NFO/PLL ==
  cos : Inport
  sin : Inport  Port=2
  Add : Sum  Inputs=-+
  Cos : Trigonometry  ApproximationMethod=Lookup
  Cos1 : Trigonometry  Operator=cos  ApproximationMethod=Lookup
  Discrete Filter2 : DiscreteFilter  Numerator=[0 0.1454]  Denominator=[1 -0.8546]
  PID Controller : slpidlib/PID Controller  Controller=PI  Form=Parallel  TimeDomain=Discrete-time  UseExternalTs=off  SampleTime=-1  IntegratorMethod=Forward Euler  FilterMethod=Forward Euler  ControllerParametersSource=internal  P=PLL_KP  I=PLL_KI  UseKiTs=off  D=0  N=100  UseFilter=on  TunerSelectOption=Transfer Function Based (PID Tuner App)  InitialConditionSource=internal  InitialConditionForIntegrator=0  InitialConditionForFilter=0  DifferentiatorICPrevScaledInput=0  ExternalReset=none  TrackingMode=off  Kt=1  LimitOutput=on  SatLimitsSource=internal  UpperSaturationLimit=3500*5/30*pi  LowerSaturationLimit=-3500*5/30*pi  LinearizeAsGain=on  AntiWindupMode=clamping  Kb=1  LimitIntegrator=off  UpperIntegratorSaturationLimit=inf  LowerIntegratorSaturationLimit=-inf  POutMin=[]  POutMax=[]  IOutMin=[]  IOutMax=[]  DOutMin=[]  DOutMax=[]  NOutMin=[]  NOutMax=[]  SumOutMin=[]  SumOutMax=[]  SaturationOutMin=[]  SaturationOutMax=[]  PParamMin=[]  PParamMax=[]  IParamMin=[]  IParamMax=[]  DParamMin=[]  DParamMax=[]  NParamMin=[]  NParamMax=[]  KbParamMin=[]  KbParamMax=[]  KtParamMin=[]  KtParamMax=[]  KbOutMin=[]  KbOutMax=[]  KtOutMin=[]  KtOutMax=[]  IntegratorOutMin=[]  IntegratorOutMax=[]  FilterOutMin=[]  FilterOutMax=[]  SumI1OutMin=[]  SumI1OutMax=[]  SumI2OutMin=[]  SumI2OutMax=[]  SumI3OutMin=[]  SumI3OutMax=[]  SumI4OutMin=[]  SumI4OutMax=[]  SumDOutMin=[]  SumDOutMax=[]  DifferentiatorOutMin=[]  DifferentiatorOutMax=[]  FilterDiffOutCoefMin=[]  FilterDiffOutCoefMax=[]  ReciprocalOutMin=[]  ReciprocalOutMax=[]  SumDenOutMin=[]  SumDenOutMax=[]  SumNumOutMin=[]  SumNumOutMax=[]  DivideOutMin=[]  DivideOutMax=[]  UdiffTsProdOutMin=[]  UdiffTsProdOutMax=[]  NTsProdOutMin=[]  NTsProdOutMax=[]  UintegralTsProdOutMin=[]  UintegralTsProdOutMax=[]  UngainTsProdOutMin=[]  UngainTsProdOutMax=[]  ClampingZeroOutDataTypeStr=Inherit: Inherit via back propagation  ClampingZeroOutMin=[]  ClampingZeroOutMax=[]  FilterDenConstantOutDataTypeStr=Inherit: Inherit via back propagation  FilterDenConstantOutMin=[]  FilterDenConstantOutMax=[]  PCopyOutDataTypeStr=Inherit: Inherit via back propagation  PCopyOutMin=[]  PCopyOutMax=[]  NCopyOutDataTypeStr=Inherit: Inherit via back propagation  NCopyOutMin=[]  NCopyOutMax=[]  IntegratorContinuousStateAttributes=''  IntegratorStateMustResolveToSignalObject=off  IntegratorRTWStateStorageClass=Auto  FilterContinuousStateAttributes=''  FilterStateMustResolveToSignalObject=off  FilterRTWStateStorageClass=Auto  ParallelPVariant=InternalParameters  IdealPVariant=Disabled  IVariant=InternalParameters  DVariant=Disabled  IntegratorVariant=Discrete  SatVariant=Enabled  AWVariant=DiscClampingParallel  PCopyVariant=Disabled  TRVariant=Disabled  FdbkBlocksVariant=Forward  IdealPFdbkVariant=Disabled  SatFdbkVariant=Disabled  DerivativeFilterVariant=Disabled  NVariant=Disabled  NCopyVariant=Disabled_SignalSpec  FilterICVariant=Disabled  IntegratorICVariant=InternalICs  ExternalResetVariant=Disabled  TRSumVariant=Passthrough  SumFdbkVariant=Disabled  SumVariant=Sum_PI  TsampFilterVariant=InternalTs  TsampNgainVariant=Passthrough  TsampIntegralVariant=Disabled_SignalSpec  ExternalSaturationOutDataTypeStr=Inherit: Same as second input
  Product : Product
  Product1 : Product
  Scope : Scope  NumInputPorts=2
  SpeedToTheta : Subsystem
  omega : Outport
  theta : Outport  Port=2
  wires:
  PID Controller/1 -> Discrete Filter2/1, SpeedToTheta/1(we)
  Add/1 -> PID Controller/1
  sin/1 -> Product1/1
  Product/1 -> Add/1
  Product1/1 -> Add/2
  Discrete Filter2/1 -> Scope/1, omega/1
  SpeedToTheta/1(Angle_output) -> Scope/2, theta/1, Cos1/1, Cos/1
  Cos/1 -> Product/2
  Cos1/1 -> Product1/2
  cos/1 -> Product/1

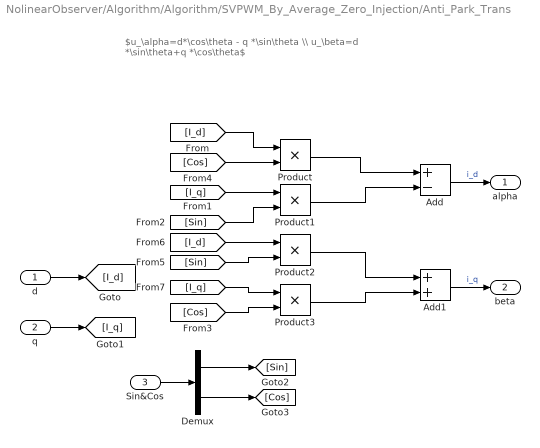
== system NolinearObserver/Algorithm/Algorithm/SVPWM_By_Average_Zero_Injection/Anti_Park_Trans ==
  note: $u_\alpha=d*\cos\theta - q *\sin\theta \\ u_\beta=d *\sin\theta+q *\cos\theta$
  d : Inport  OutDataTypeStr=single
  q : Inport  Port=2  OutDataTypeStr=single
  Sin&Cos : Inport  Port=3  OutDataTypeStr=single
  Add : Sum  Inputs=+-  OutDataTypeStr=single
  Add1 : Sum  OutDataTypeStr=single
  Demux : Demux  Outputs=2
  Product{,1..3} (4 alike) : Product  OutDataTypeStr=single
  alpha : Outport  OutDataTypeStr=single
  beta : Outport  Port=2  OutDataTypeStr=single
  wires:
  Add1/1 -> beta/1  "i_q"
  Sin&Cos/1 -> Demux/1
  [Cos] -> Product/2
  Product/1 -> Add/1
  Product1/1 -> Add/2
  q/1 -> [I_q]
  Add/1 -> alpha/1  "i_d"
  [I_d] -> Product/1
  Product3/1 -> Add1/2
  [I_q] -> Product3/1
  [I_q] -> Product1/1
  [Sin] -> Product2/2
  Product2/1 -> Add1/1
  [Sin] -> Product1/2
  [I_d] -> Product2/1
  d/1 -> [I_d]
  [Cos] -> Product3/2
  Demux/1 -> [Sin]
  Demux/2 -> [Cos]

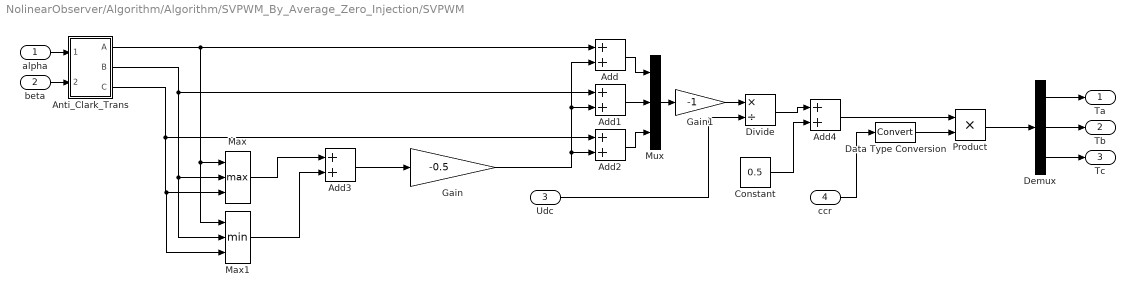
== system NolinearObserver/Algorithm/Algorithm/SVPWM_By_Average_Zero_Injection/SVPWM ==
  alpha : Inport  OutDataTypeStr=single
  beta : Inport  Port=2  OutDataTypeStr=single
  Udc : Inport  Port=3  OutDataTypeStr=single
  ccr : Inport  Port=4
  Add{,1..4} (5 alike) : Sum  OutDataTypeStr=single
  Anti_Clark_Trans : Subsystem
  Constant : Constant  Value=0.5  OutDataTypeStr=single  SampleTime=Ts
  Data Type Conversion : DataTypeConversion  SaturateOnIntegerOverflow=off  RndMeth=Floor
  Demux : Demux  Outputs=3
  Divide : Product  Inputs=*/  OutDataTypeStr=single
  Gain : Gain  Gain=-0.5  OutDataTypeStr=single
  Gain1 : Gain  Gain=-1  OutDataTypeStr=single
  Max : MinMax  Function=max  Inputs=3  OutDataTypeStr=single
  Max1 : MinMax  Inputs=3  OutDataTypeStr=single
  Mux : Mux  Inputs=3
  Product : Product
  Ta : Outport  OutDataTypeStr=single
  Tb : Outport  Port=2  OutDataTypeStr=single
  Tc : Outport  Port=3  OutDataTypeStr=single
  wires:
  Anti_Clark_Trans/1(A) -> Max1/1, Max/1, Add/1
  Gain/1 -> Add/2, Add1/2, Add2/2
  Anti_Clark_Trans/2(B) -> Max1/2, Max/2, Add1/1
  Anti_Clark_Trans/3(C) -> Max1/3, Max/3, Add2/1
  Add3/1 -> Gain/1
  Max/1 -> Add3/1
  alpha/1 -> Anti_Clark_Trans/1(alpha)
  beta/1 -> Anti_Clark_Trans/2(beta)
  Add/1 -> Mux/1
  Add1/1 -> Mux/2
  Add2/1 -> Mux/3
  Demux/1 -> Ta/1
  Demux/2 -> Tb/1
  Demux/3 -> Tc/1
  Divide/1 -> Add4/1
  Constant/1 -> Add4/2
  Max1/1 -> Add3/2
  Udc/1 -> Divide/2
  Mux/1 -> Gain1/1
  Gain1/1 -> Divide/1
  Add4/1 -> Product/1
  Product/1 -> Demux/1
  ccr/1 -> Data Type Conversion/1
  Data Type Conversion/1 -> Product/2

== system NolinearObserver/Algorithm/Algorithm/IF_Switch_Logical/Forward_theta/integrator/RangeLimit ==
  In : Inport  OutDataTypeStr=single
  Constant : Constant  Value=2*pi  OutDataTypeStr=single  SampleTime=-1
  Constant1 : Constant  Value=0  OutDataTypeStr=single  SampleTime=-1
  If : If  NumInputs=2  IfExpression=u1  ElseIfExpressions=u2
  If Action Subsystem : Subsystem  TreatAsAtomicUnit=on
  If Action Subsystem1 : Subsystem  TreatAsAtomicUnit=on
  If Action Subsystem2 : Subsystem  TreatAsAtomicUnit=on
  Merge : Merge  Inputs=3
  Relational Operator : RelationalOperator  Operator=>  OutDataTypeStr=boolean  RndMeth=Simplest  InputSameDT=off
  Relational Operator1 : RelationalOperator  Operator=<  OutDataTypeStr=boolean  RndMeth=Simplest  InputSameDT=off
  Theta : Outport  OutDataTypeStr=single
  wires:
  Relational Operator/1 -> If/1
  Constant/1 -> Relational Operator/2
  Constant1/1 -> Relational Operator1/2
  In/1 -> Relational Operator1/1, If Action Subsystem2/1(In1), If Action Subsystem1/1(In1), If Action Subsystem/1(In1), Relational Operator/1
  Relational Operator1/1 -> If/2
  Merge/1 -> Theta/1
  If/3 -> If Action Subsystem2/Action
  If/2 -> If Action Subsystem/Action
  If/1 -> If Action Subsystem1/Action
  If Action Subsystem2/1(Out1) -> Merge/1
  If Action Subsystem/1(Out1) -> Merge/2
  If Action Subsystem1/1(Out1) -> Merge/3

== system NolinearObserver/Algorithm/Algorithm/NFO/PLL/SpeedToTheta ==
  we : Inport
  Angle_Limit : Subsystem
  Data Type Conversion : DataTypeConversion  SaturateOnIntegerOverflow=off  RndMeth=Floor
  Data Type Conversion1 : DataTypeConversion  SaturateOnIntegerOverflow=off  RndMeth=Floor
  Gain : Gain  Gain=Ts
  Sum : Sum  Inputs=|++
  Unit Delay : UnitDelay  SampleTime=-1  HasFrameUpgradeWarning=on
  Angle_output : Outport
  wires:
  we/1 -> Gain/1
  Gain/1 -> Sum/1
  Unit Delay/1 -> Sum/2, Angle_output/1
  Angle_Limit/1(Angle_output) -> Data Type Conversion/1
  Data Type Conversion/1 -> Unit Delay/1
  Data Type Conversion1/1 -> Angle_Limit/1(Angle_input)
  Sum/1 -> Data Type Conversion1/1

== system NolinearObserver/Algorithm/Algorithm/SVPWM_By_Average_Zero_Injection/SVPWM/Anti_Clark_Trans ==
  alpha : Inport  OutDataTypeStr=single
  beta : Inport  Port=2  OutDataTypeStr=single
  Add : Sum  Inputs=-+  OutDataTypeStr=single
  Add1 : Sum  Inputs=--  OutDataTypeStr=single
  Gain : Gain  Gain=0.5  OutDataTypeStr=single
  Gain1 : Gain  Gain=sqrt(3)/2  OutDataTypeStr=single
  A : Outport  OutDataTypeStr=single
  B : Outport  Port=2  OutDataTypeStr=single
  C : Outport  Port=3  OutDataTypeStr=single
  wires:
  Add1/1 -> C/1
  Gain/1 -> Add1/1, Add/1
  Add/1 -> B/1
  alpha/1 -> A/1, Gain/1
  Gain1/1 -> Add1/2, Add/2
  beta/1 -> Gain1/1

== system NolinearObserver/Algorithm/Algorithm/IF_Switch_Logical/Forward_theta/integrator/RangeLimit/If Action Subsystem ==
  In1 : Inport  OutDataTypeStr=single
  Action Port : ActionPort  ActionPortLabel=elseif(u2)
  Constant : Constant  Value=2*pi  OutDataTypeStr=single  SampleTime=-1
  Sum : Sum  Inputs=|++  OutDataTypeStr=single
  Out1 : Outport  OutDataTypeStr=single
  wires:
  In1/1 -> Sum/1
  Constant/1 -> Sum/2
  Sum/1 -> Out1/1

== system NolinearObserver/Algorithm/Algorithm/IF_Switch_Logical/Forward_theta/integrator/RangeLimit/If Action Subsystem1 ==
  In1 : Inport  OutDataTypeStr=single
  Action Port : ActionPort  ActionPortLabel=if(u1)
  Constant : Constant  Value=2*pi  OutDataTypeStr=single  SampleTime=-1
  Sum : Sum  Inputs=|+-  OutDataTypeStr=single
  Out1 : Outport  OutDataTypeStr=single
  wires:
  In1/1 -> Sum/1
  Constant/1 -> Sum/2
  Sum/1 -> Out1/1

== system NolinearObserver/Algorithm/Algorithm/IF_Switch_Logical/Forward_theta/integrator/RangeLimit/If Action Subsystem2 ==
  In1 : Inport  OutDataTypeStr=single
  Action Port : ActionPort  ActionPortLabel=else
  Out1 : Outport  OutDataTypeStr=single
  wires:
  In1/1 -> Out1/1

== system NolinearObserver/Algorithm/Algorithm/NFO/PLL/SpeedToTheta/Angle_Limit ==
  Angle_input : Inport
  If : If  IfExpression=u1 > 6.28318307  ElseIfExpressions=u1 < 0
  If Action Subsystem : Subsystem  TreatAsAtomicUnit=on
  If Action Subsystem1 : Subsystem  TreatAsAtomicUnit=on
  If Action Subsystem2 : Subsystem  TreatAsAtomicUnit=on
  Merge : Merge  Inputs=3
  Angle_output : Outport
  wires:
  Angle_input/1 -> If Action Subsystem2/1(Angle_input), If Action Subsystem1/1(Angle_input), If Action Subsystem/1(Angle_input), If/1
  If/1 -> If Action Subsystem/Action
  If/2 -> If Action Subsystem1/Action
  If/3 -> If Action Subsystem2/Action
  Merge/1 -> Angle_output/1
  If Action Subsystem1/1(Out1) -> Merge/2
  If Action Subsystem/1(Out1) -> Merge/1
  If Action Subsystem2/1(Out1) -> Merge/3

== system NolinearObserver/Algorithm/Algorithm/NFO/PLL/SpeedToTheta/Angle_Limit/If Action Subsystem ==
  Angle_input : Inport
  Action Port : ActionPort  ActionPortLabel=if(u1 > 6.28318307)
  Add : Sum  Inputs=+-
  Constant : Constant  Value=6.28318307
  Out1 : Outport
  wires:
  Angle_input/1 -> Add/1
  Add/1 -> Out1/1
  Constant/1 -> Add/2

== system NolinearObserver/Algorithm/Algorithm/NFO/PLL/SpeedToTheta/Angle_Limit/If Action Subsystem1 ==
  Angle_input : Inport
  Action Port : ActionPort  ActionPortLabel=elseif(u1 < 0)
  Add : Sum
  Constant : Constant  Value=6.28318307
  Out1 : Outport
  wires:
  Angle_input/1 -> Add/1
  Add/1 -> Out1/1
  Constant/1 -> Add/2

== system NolinearObserver/Algorithm/Algorithm/NFO/PLL/SpeedToTheta/Angle_Limit/If Action Subsystem2 ==
  Angle_input : Inport
  Action Port : ActionPort  ActionPortLabel=else
  Out1 : Outport
  wires:
  Angle_input/1 -> Out1/1

== stateflow chart NolinearObserver/Algorithm/Chart1 ==
  state Out = Over_judge(Input) [function]
  state Out = Low_judge(Input) [function]
  state None
    during:
    Over_V= Over_judge(Udc);
    Low_V= Low_judge(Udc);
    STOP=Low_V+Over_V;
    exit:
    Over_V= Over_judge(Udc);
    Low_V= Low_judge(Udc);
    STOP=Low_V+Over_V;
  state Out
    during:
    Over_V=Over_judge(Udc);
    Low_V= Low_judge(Udc);
    STOP=Low_V+Over_V;
    Go = 1;
  (default) -> None : {up_limit = 28;down_limit = 15;}
  None -> Out : [Go_Flag == 1 && STOP ==0 ]
  Out -> None [order 2] : [Go_Flag == 0 ]
  Out -> None [order 1] : [ Over_V ==1|| Low_V==1]{Go = 0}
  data: Input function_input single size=1; Out function_output single; Input function_input single size=1; Out function_output single; Go_Flag input; Udc input; Over_V output single size=1 =0; STOP output single =0; Low_V output single size=1 =0; down_limit local; up_limit local; Go output =0

== stateflow chart NolinearObserver/Algorithm/Algorithm/IF_Switch_Logical ==
  state Forward
    [IF_theta,omega_IF]=Forward_theta(direction);
    error_theta=Obe_theta-IF_theta;
    iqavg=Iq_set_in*cos(error_theta) ;
    state tcos_state1
      tcos=single(1);
      Iq_out=Iq_set_in;
      Use_Theta=tcos*IF_theta + (1-tcos)*Obe_theta;
    state tcos_state2
      tcos=cos((abs(omega_IF) -omega1)/(omega2-omega1)*pi/2);
      Iq_out=iqavg/cos(tcos*error_theta);
      Use_Theta=tcos*IF_theta + (1-tcos)*Obe_theta;
      Iq_keep=Iq_out;
    state Swich_over
      enable=single(1);
      Iq_out=Iq_keep;
      Use_Theta=Obe_theta;
    (default) -> Forward.tcos_state1 : {Iq_keep=0;}
    Forward.tcos_state1 -> Forward.tcos_state2 : [omega1<abs(omega_IF) && abs(omega_IF) <omega2]
    Forward.tcos_state2 -> Forward.Swich_over : [abs(omega_IF) >=omega2]
  state [IF_theta,IF_omega] = Forward_theta(direction) [function]
  state Speed_interve
    Iq_out=Speed_set_in;
    Use_Theta=Obe_theta;
  state direction_judge
    (default) -> (junction 14) : % direction_judge
    (junction 14) -> (junction 15) [order 1] : [Ref_RPM > 30]
    (junction 14) -> (junction 16) [order 2]
    (junction 15) -> (junction 20) : {direction = 1;}
    (junction 16) -> (junction 17) [order 1] : [Ref_RPM < -30]
    (junction 16) -> (junction 18) [order 2]
    (junction 17) -> (junction 19) : {direction = -1;}
    (junction 19) -> (junction 18)
    (junction 20) -> (junction 19)
    (junction 18) -> (junction 21)
  state Backward
    [IF_theta,omega_IF]=Forward_theta(direction);
    error_theta=Obe_theta-IF_theta;
    iqavg=Iq_set_in*cos(error_theta) ;
    state tcos_state1
      tcos=single(1);
      Iq_out=Iq_set_in;
      Use_Theta=tcos*IF_theta + (1-tcos)*Obe_theta;
    state tcos_state2
      tcos=cos((abs(omega_IF) -omega1)/(omega2-omega1)*pi/2);
      Iq_out=iqavg/cos(tcos*error_theta);
      Use_Theta=tcos*IF_theta + (1-tcos)*Obe_theta;
      Iq_keep=Iq_out;
    state Swich_over
      Iq_out=Iq_keep;
      Use_Theta=Obe_theta;
      enable=single(1);
    (default) -> Backward.tcos_state1 : {Iq_keep=0;}
    Backward.tcos_state1 -> Backward.tcos_state2 : [omega1<abs(omega_IF) && abs(omega_IF) <omega2]
    Backward.tcos_state2 -> Backward.Swich_over : [abs(omega_IF) >=omega2]
  state Speed_interve1
    Iq_out=Speed_set_in;
    Use_Theta=Obe_theta;
  Forward -> Speed_interve : [ enable ==1 && Speed_set_in > Iq_keep ]
  (default) -> direction_judge : {omega1=single(80);omega2=single(81);}
  direction_judge -> Forward [order 1] : [direction==1]
  Backward -> Speed_interve1 : [enable ==1 && Speed_set_in < Iq_keep]
  direction_judge -> Backward [order 2] : [direction==-1]
  data: IF_theta function_output single; IF_omega function_output single; direction function_input single size=1; Ref_RPM input single; direction local single; Use_Theta output single; Iq_out output single; Iq_set_in input single; Speed_set_in input single; Obe_theta input single; enable output single =0; iqavg local single =0; omega1 local single; omega2 local single; IF_theta local single; tcos output single; error_theta local single; omega_IF output single; Iq_keep local single
